simulink subsystem "Motores"  (R2023b)
settings: Solver=VariableStepAuto  StartTime=0.0  StopTime=10.0  RelTol=1e-3
libraries: arduinolib x4
settings Model: Creator=Andrés  LastModifiedBy=Andrés

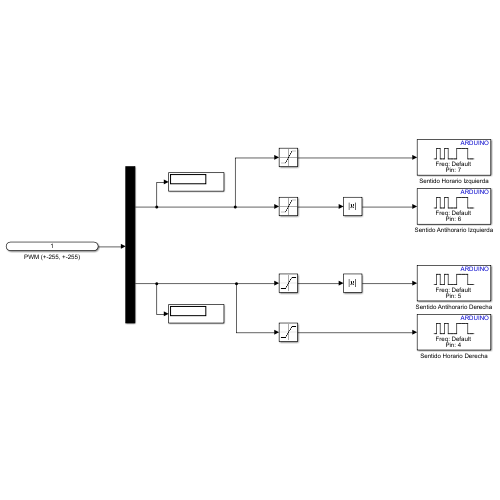
[thumbnail: Simulink's stored preview of the top-level diagram]
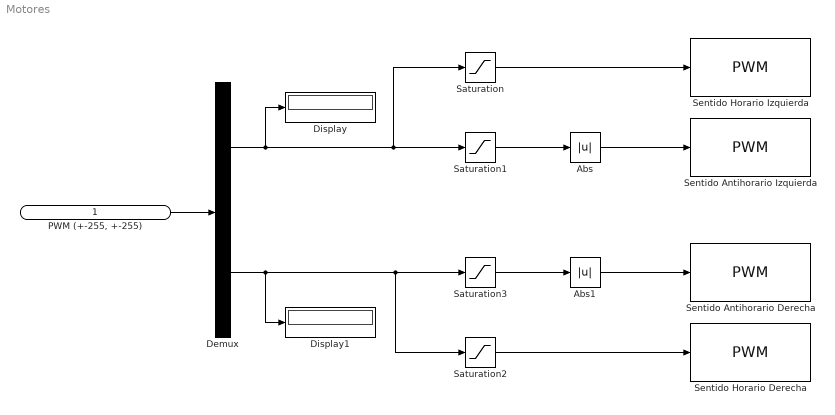
== system Motores ==
  "PWM (+-255, +-255)" : Inport
  Abs : Abs  SaturateOnIntegerOverflow=off
  Abs1 : Abs  SaturateOnIntegerOverflow=off
  Demux : Demux  Outputs=2
  Display : Display
  Display1 : Display
  Saturation : Saturate  UpperLimit=255  LowerLimit=0
  Saturation1 : Saturate  UpperLimit=0  LowerLimit=-255
  Saturation2 : Saturate  UpperLimit=255  LowerLimit=0
  Saturation3 : Saturate  UpperLimit=0  LowerLimit=-255
  Sentido Antihorario Derecha : arduinolib/PWM  pinNumber=5  frequencyType=Default  desiredFrequency=490.2  achievableFrequency=490.2
  Sentido Antihorario Izquierda : arduinolib/PWM  pinNumber=6  frequencyType=Default  desiredFrequency=490.2  achievableFrequency=490.2
  Sentido Horario Derecha : arduinolib/PWM  pinNumber=4  frequencyType=Default  desiredFrequency=490.2  achievableFrequency=490.2
  Sentido Horario Izquierda : arduinolib/PWM  pinNumber=7  frequencyType=Default  desiredFrequency=490.2  achievableFrequency=490.2
  wires:
  Demux/2 -> Display1/1, Saturation3/1, Saturation2/1
  Abs1/1 -> Sentido Antihorario Derecha/1
  Saturation/1 -> Sentido Horario Izquierda/1
  Saturation2/1 -> Sentido Horario Derecha/1
  Abs/1 -> Sentido Antihorario Izquierda/1
  Demux/1 -> Saturation1/1, Saturation/1, Display/1
  Saturation1/1 -> Abs/1
  "PWM (+-255, +-255)"/1 -> Demux/1
  Saturation3/1 -> Abs1/1
